simulink library "PUD_lib"  (Simulink 7.5)
settings: Solver=ode45  StartTime=0.0  StopTime=10.0  RelTol=1e-3
values from neighbouring files (symbols this model uses):
  pPUD_cnt_ACChItErrThd_C = Simulink.Parameter    [PUD_par.m]
  pPUD_cnt_ACHeatItErrThd_C = Simulink.Parameter    [PUD_par.m]
  pPUD_cnt_DCChItErrThd_C = Simulink.Parameter    [PUD_par.m]
  pPUD_cnt_DCHeatItErrThd_C = Simulink.Parameter    [PUD_par.m]
  pPUD_s_ACChrg1NoRespTiout_C = Simulink.Parameter    [PUD_par.m]
  pPUD_s_ACChrg2NoRespTiout_C = Simulink.Parameter    [PUD_par.m]
  pPUD_s_ACChrgPtcEnDly_C = Simulink.Parameter    [PUD_par.m]
  pPUD_s_BMSOnNoRespTiout_C = Simulink.Parameter    [PUD_par.m]
  pPUD_s_DCChrg1NoRespTiout_C = Simulink.Parameter    [PUD_par.m]
  pPUD_s_DCChrg2NoRespTiout_C = Simulink.Parameter    [PUD_par.m]
  pPUD_s_EgyCoorrChItRecoverDly_C = Simulink.Parameter    [PUD_par.m]
  pPUD_s_EgyCoorrDlyRstCtr_C = Simulink.Parameter    [PUD_par.m]
  pPUD_s_EgyCoorrNoRespTiout_C = Simulink.Parameter    [PUD_par.m]
  pPUD_V_MotPwrVolt_C = Simulink.Parameter    [PUD_par.m]
  pPUD_V_MotRpdDisVolt_C = Simulink.Parameter    [PUD_par.m]
libraries: BaseOperationLib_Browser x22, PES_CZ_FAW x7, simulink x1
settings Model: Creator=wuaibin  LastModifiedBy=wuaibin

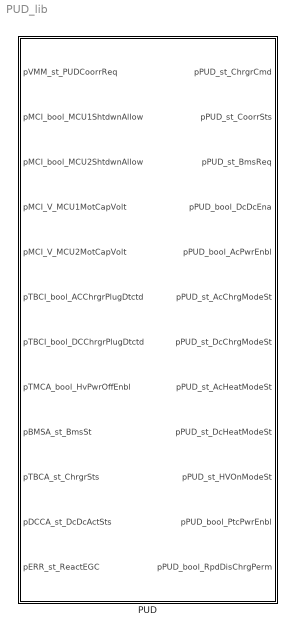
== system PUD_lib ==
  PUD : Subsystem  TreatAsAtomicUnit=on

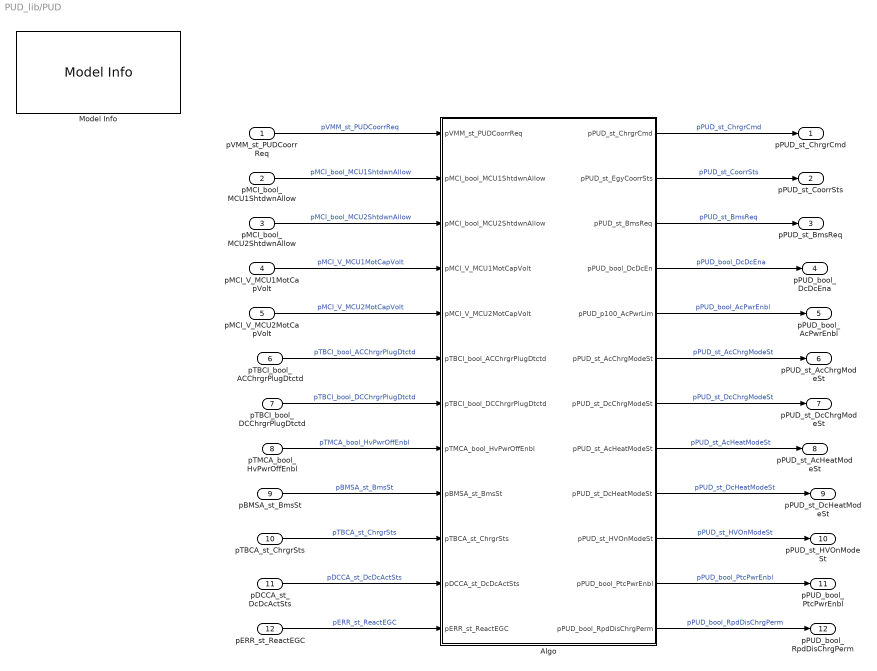
== system PUD_lib/PUD ==
  pVMM_st_PUDCoorrReq : Inport
  pMCI_bool_MCU1ShtdwnAllow : Inport  Port=2
  pMCI_bool_MCU2ShtdwnAllow : Inport  Port=3
  pMCI_V_MCU1MotCapVolt : Inport  Port=4
  pMCI_V_MCU2MotCapVolt : Inport  Port=5
  pTBCI_bool_ACChrgrPlugDtctd : Inport  Port=6
  pTBCI_bool_DCChrgrPlugDtctd : Inport  Port=7
  pTMCA_bool_HvPwrOffEnbl : Inport  Port=8
  pBMSA_st_BmsSt : Inport  Port=9
  pTBCA_st_ChrgrSts : Inport  Port=10
  pDCCA_st_DcDcActSts : Inport  Port=11
  pERR_st_ReactEGC : Inport  Port=12
  Algo : Subsystem
  Model Info : simulink/Model-Wide Utilities/Model Info  SystemSampleTime=-1  InitialBlockCM=None  BlockCM=None  Frame=on  DisplayStringWithTags=Model Info\nCreated: %<Created>\nCreator: wuaibin  HorizontalTextAlignment=Center  LeftAlignmentValue=0.5  SourceBlockDiagram=HQEV_HCU  TagMaxNumber=20
  pPUD_st_ChrgrCmd : Outport
  pPUD_st_CoorrSts : Outport  Port=2
  pPUD_st_BmsReq : Outport  Port=3
  pPUD_bool_DcDcEna : Outport  Port=4
  pPUD_bool_AcPwrEnbl : Outport  Port=5
  pPUD_st_AcChrgModeSt : Outport  Port=6
  pPUD_st_DcChrgModeSt : Outport  Port=7
  pPUD_st_AcHeatModeSt : Outport  Port=8
  pPUD_st_DcHeatModeSt : Outport  Port=9
  pPUD_st_HVOnModeSt : Outport  Port=10
  pPUD_bool_PtcPwrEnbl : Outport  Port=11
  pPUD_bool_RpdDisChrgPerm : Outport  Port=12
  wires:
  pERR_st_ReactEGC/1 -> Algo/12(pERR_st_ReactEGC)  "pERR_st_ReactEGC"
  Algo/12(pPUD_bool_RpdDisChrgPerm) -> pPUD_bool_RpdDisChrgPerm/1  "pPUD_bool_RpdDisChrgPerm"
  pMCI_V_MCU2MotCapVolt/1 -> Algo/5(pMCI_V_MCU2MotCapVolt)  "pMCI_V_MCU2MotCapVolt"
  pMCI_V_MCU1MotCapVolt/1 -> Algo/4(pMCI_V_MCU1MotCapVolt)  "pMCI_V_MCU1MotCapVolt"
  Algo/11(pPUD_bool_PtcPwrEnbl) -> pPUD_bool_PtcPwrEnbl/1  "pPUD_bool_PtcPwrEnbl"
  Algo/10(pPUD_st_HVOnModeSt) -> pPUD_st_HVOnModeSt/1  "pPUD_st_HVOnModeSt"
  Algo/9(pPUD_st_DcHeatModeSt) -> pPUD_st_DcHeatModeSt/1  "pPUD_st_DcHeatModeSt"
  Algo/8(pPUD_st_AcHeatModeSt) -> pPUD_st_AcHeatModeSt/1  "pPUD_st_AcHeatModeSt"
  Algo/7(pPUD_st_DcChrgModeSt) -> pPUD_st_DcChrgModeSt/1  "pPUD_st_DcChrgModeSt"
  Algo/6(pPUD_st_AcChrgModeSt) -> pPUD_st_AcChrgModeSt/1  "pPUD_st_AcChrgModeSt"
  Algo/5(pPUD_p100_AcPwrLim) -> pPUD_bool_AcPwrEnbl/1  "pPUD_bool_AcPwrEnbl"
  Algo/4(pPUD_bool_DcDcEn) -> pPUD_bool_DcDcEna/1  "pPUD_bool_DcDcEna"
  Algo/3(pPUD_st_BmsReq) -> pPUD_st_BmsReq/1  "pPUD_st_BmsReq"
  Algo/2(pPUD_st_EgyCoorrSts) -> pPUD_st_CoorrSts/1  "pPUD_st_CoorrSts"
  Algo/1(pPUD_st_ChrgrCmd) -> pPUD_st_ChrgrCmd/1  "pPUD_st_ChrgrCmd"
  pDCCA_st_DcDcActSts/1 -> Algo/11(pDCCA_st_DcDcActSts)  "pDCCA_st_DcDcActSts"
  pTBCA_st_ChrgrSts/1 -> Algo/10(pTBCA_st_ChrgrSts)  "pTBCA_st_ChrgrSts"
  pBMSA_st_BmsSt/1 -> Algo/9(pBMSA_st_BmsSt)  "pBMSA_st_BmsSt"
  pTMCA_bool_HvPwrOffEnbl/1 -> Algo/8(pTMCA_bool_HvPwrOffEnbl)  "pTMCA_bool_HvPwrOffEnbl"
  pMCI_bool_MCU2ShtdwnAllow/1 -> Algo/3(pMCI_bool_MCU2ShtdwnAllow)  "pMCI_bool_MCU2ShtdwnAllow"
  pMCI_bool_MCU1ShtdwnAllow/1 -> Algo/2(pMCI_bool_MCU1ShtdwnAllow)  "pMCI_bool_MCU1ShtdwnAllow"
  pVMM_st_PUDCoorrReq/1 -> Algo/1(pVMM_st_PUDCoorrReq)  "pVMM_st_PUDCoorrReq"
  pTBCI_bool_ACChrgrPlugDtctd/1 -> Algo/6(pTBCI_bool_ACChrgrPlugDtctd)  "pTBCI_bool_ACChrgrPlugDtctd"
  pTBCI_bool_DCChrgrPlugDtctd/1 -> Algo/7(pTBCI_bool_DCChrgrPlugDtctd)  "pTBCI_bool_DCChrgrPlugDtctd"

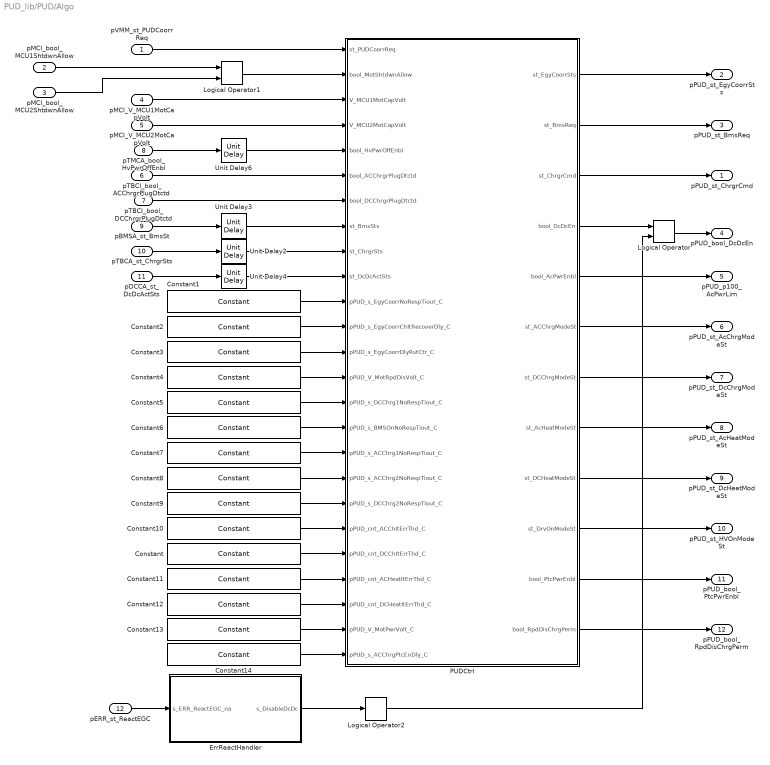
== system PUD_lib/PUD/Algo ==
  pVMM_st_PUDCoorrReq : Inport
  pMCI_bool_MCU1ShtdwnAllow : Inport  Port=2
  pMCI_bool_MCU2ShtdwnAllow : Inport  Port=3
  pMCI_V_MCU1MotCapVolt : Inport  Port=4
  pMCI_V_MCU2MotCapVolt : Inport  Port=5
  pTBCI_bool_ACChrgrPlugDtctd : Inport  Port=6
  pTBCI_bool_DCChrgrPlugDtctd : Inport  Port=7
  pTMCA_bool_HvPwrOffEnbl : Inport  Port=8
  pBMSA_st_BmsSt : Inport  Port=9
  pTBCA_st_ChrgrSts : Inport  Port=10
  pDCCA_st_DcDcActSts : Inport  Port=11
  pERR_st_ReactEGC : Inport  Port=12
  Constant : BaseOperationLib_Browser/Sources&Sinks/Constant  Value=pPUD_cnt_DCChItErrThd_C  OutMin=[]  OutMax=[]  OutDataType=fixdt(1, 16)  ConRadixGroup=Use specified scaling  OutScaling=2^0  OutDataTypeStr=Inherit: Inherit from 'Constant value'
  Constant1 : BaseOperationLib_Browser/Sources&Sinks/Constant  Value=pPUD_s_EgyCoorrNoRespTiout_C  OutMin=[]  OutMax=[]  OutDataType=fixdt(1, 16)  ConRadixGroup=Use specified scaling  OutScaling=2^0  OutDataTypeStr=Inherit: Inherit from 'Constant value'
  Constant10 : BaseOperationLib_Browser/Sources&Sinks/Constant  Value=pPUD_cnt_ACChItErrThd_C  OutMin=[]  OutMax=[]  OutDataType=fixdt(1, 16)  ConRadixGroup=Use specified scaling  OutScaling=2^0  OutDataTypeStr=Inherit: Inherit from 'Constant value'
  Constant11 : BaseOperationLib_Browser/Sources&Sinks/Constant  Value=pPUD_cnt_ACHeatItErrThd_C  OutMin=[]  OutMax=[]  OutDataType=fixdt(1, 16)  ConRadixGroup=Use specified scaling  OutScaling=2^0  OutDataTypeStr=Inherit: Inherit from 'Constant value'
  Constant12 : BaseOperationLib_Browser/Sources&Sinks/Constant  Value=pPUD_cnt_DCHeatItErrThd_C  OutMin=[]  OutMax=[]  OutDataType=fixdt(1, 16)  ConRadixGroup=Use specified scaling  OutScaling=2^0  OutDataTypeStr=Inherit: Inherit from 'Constant value'
  Constant13 : BaseOperationLib_Browser/Sources&Sinks/Constant  Value=pPUD_V_MotPwrVolt_C  OutMin=[]  OutMax=[]  OutDataType=fixdt(1, 16)  ConRadixGroup=Use specified scaling  OutScaling=2^0  OutDataTypeStr=Inherit: Inherit from 'Constant value'
  Constant14 : BaseOperationLib_Browser/Sources&Sinks/Constant  Value=pPUD_s_ACChrgPtcEnDly_C  OutMin=[]  OutMax=[]  OutDataType=fixdt(1, 16)  ConRadixGroup=Use specified scaling  OutScaling=2^0  OutDataTypeStr=Inherit: Inherit from 'Constant value'
  Constant2 : BaseOperationLib_Browser/Sources&Sinks/Constant  Value=pPUD_s_EgyCoorrChItRecoverDly_C  OutMin=[]  OutMax=[]  OutDataType=fixdt(1, 16)  ConRadixGroup=Use specified scaling  OutScaling=2^0  OutDataTypeStr=Inherit: Inherit from 'Constant value'
  Constant3 : BaseOperationLib_Browser/Sources&Sinks/Constant  Value=pPUD_s_EgyCoorrDlyRstCtr_C  OutMin=[]  OutMax=[]  OutDataType=fixdt(1, 16)  ConRadixGroup=Use specified scaling  OutScaling=2^0  OutDataTypeStr=Inherit: Inherit from 'Constant value'
  Constant4 : BaseOperationLib_Browser/Sources&Sinks/Constant  Value=pPUD_V_MotRpdDisVolt_C  OutMin=[]  OutMax=[]  OutDataType=fixdt(1, 16)  ConRadixGroup=Use specified scaling  OutScaling=2^0  OutDataTypeStr=Inherit: Inherit from 'Constant value'
  Constant5 : BaseOperationLib_Browser/Sources&Sinks/Constant  Value=pPUD_s_DCChrg1NoRespTiout_C  OutMin=[]  OutMax=[]  OutDataType=fixdt(1, 16)  ConRadixGroup=Use specified scaling  OutScaling=2^0  OutDataTypeStr=Inherit: Inherit from 'Constant value'
  Constant6 : BaseOperationLib_Browser/Sources&Sinks/Constant  Value=pPUD_s_BMSOnNoRespTiout_C  VectorParams1D=off  OutMin=[]  OutMax=[]  OutDataType=fixdt(1, 16)  ConRadixGroup=Use specified scaling  OutScaling=2^0  OutDataTypeStr=Inherit: Inherit from 'Constant value'
  Constant7 : BaseOperationLib_Browser/Sources&Sinks/Constant  Value=pPUD_s_ACChrg1NoRespTiout_C  OutMin=[]  OutMax=[]  OutDataType=fixdt(1, 16)  ConRadixGroup=Use specified scaling  OutScaling=2^0  OutDataTypeStr=Inherit: Inherit from 'Constant value'
  Constant8 : BaseOperationLib_Browser/Sources&Sinks/Constant  Value=pPUD_s_ACChrg2NoRespTiout_C  OutMin=[]  OutMax=[]  OutDataType=fixdt(1, 16)  ConRadixGroup=Use specified scaling  OutScaling=2^0  OutDataTypeStr=Inherit: Inherit from 'Constant value'
  Constant9 : BaseOperationLib_Browser/Sources&Sinks/Constant  Value=pPUD_s_DCChrg2NoRespTiout_C  OutMin=[]  OutMax=[]  OutDataType=fixdt(1, 16)  ConRadixGroup=Use specified scaling  OutScaling=2^0  OutDataTypeStr=Inherit: Inherit from 'Constant value'
  ErrReactHandler : Subsystem
  Logical Operator : BaseOperationLib_Browser/Logic Operations Changed/Logical Operator  Operator=AND  Inputs=2  AllPortsSameDT=off  OutDataTypeMode=boolean  LogicDataType=PDT_Bool  OutDataTypeStr=boolean
  Logical Operator1 : BaseOperationLib_Browser/Logic Operations Changed/Logical Operator  Operator=AND  Inputs=2  AllPortsSameDT=off  OutDataTypeMode=boolean  LogicDataType=PDT_Bool  OutDataTypeStr=boolean
  Logical Operator2 : BaseOperationLib_Browser/Logic Operations Changed/Logical Operator  Operator=NOT  Inputs=2  AllPortsSameDT=off  OutDataTypeMode=boolean  LogicDataType=PDT_Bool  OutDataTypeStr=boolean
  PUDCtrl : Stateflow chart  TreatAsAtomicUnit=on
  Unit Delay{2..4,6} (4 alike) : BaseOperationLib_Browser/Discrete Unchanged /Unit Delay  X0=0  SampleTime=-1
  pPUD_st_ChrgrCmd : Outport
  pPUD_st_EgyCoorrSts : Outport  Port=2
  pPUD_st_BmsReq : Outport  Port=3
  pPUD_bool_DcDcEn : Outport  Port=4
  pPUD_p100_AcPwrLim : Outport  Port=5
  pPUD_st_AcChrgModeSt : Outport  Port=6
  pPUD_st_DcChrgModeSt : Outport  Port=7
  pPUD_st_AcHeatModeSt : Outport  Port=8
  pPUD_st_DcHeatModeSt : Outport  Port=9
  pPUD_st_HVOnModeSt : Outport  Port=10
  pPUD_bool_PtcPwrEnbl : Outport  Port=11
  pPUD_bool_RpdDisChrgPerm : Outport  Port=12
  wires:
  Logical Operator2/1 -> Logical Operator/2
  Constant12/1 -> PUDCtrl/23(pPUD_cnt_DCHeatItErrThd_C)
  Constant11/1 -> PUDCtrl/22(pPUD_cnt_ACHeatItErrThd_C)
  Constant10/1 -> PUDCtrl/20(pPUD_cnt_ACChItErrThd_C)
  Constant9/1 -> PUDCtrl/19(pPUD_s_DCChrg2NoRespTiout_C)
  Constant8/1 -> PUDCtrl/18(pPUD_s_ACChrg2NoRespTiout_C)
  Constant7/1 -> PUDCtrl/17(pPUD_s_ACChrg1NoRespTiout_C)
  Constant6/1 -> PUDCtrl/16(pPUD_s_BMSOnNoRespTiout_C)
  Constant5/1 -> PUDCtrl/15(pPUD_s_DCChrg1NoRespTiout_C)
  Constant4/1 -> PUDCtrl/14(pPUD_V_MotRpdDisVolt_C)
  Constant3/1 -> PUDCtrl/13(pPUD_s_EgyCoorrDlyRstCtr_C)
  Constant2/1 -> PUDCtrl/12(pPUD_s_EgyCoorrChItRecoverDly_C)
  Constant1/1 -> PUDCtrl/11(pPUD_s_EgyCoorrNoRespTiout_C)
  Constant/1 -> PUDCtrl/21(pPUD_cnt_DCChItErrThd_C)
  pERR_st_ReactEGC/1 -> ErrReactHandler/1(s_ERR_ReactEGC_na)
  ErrReactHandler/1(s_DisableDcDc) -> Logical Operator2/1
  Logical Operator/1 -> pPUD_bool_DcDcEn/1
  PUDCtrl/12(bool_RpdDisChrgPerm) -> pPUD_bool_RpdDisChrgPerm/1
  pMCI_V_MCU2MotCapVolt/1 -> PUDCtrl/4(V_MCU2MotCapVolt)
  pMCI_V_MCU1MotCapVolt/1 -> PUDCtrl/3(V_MCU1MotCapVolt)
  Logical Operator1/1 -> PUDCtrl/2(bool_MotShtdwnAllow)
  pMCI_bool_MCU1ShtdwnAllow/1 -> Logical Operator1/1
  pMCI_bool_MCU2ShtdwnAllow/1 -> Logical Operator1/2
  Unit Delay4/1 -> PUDCtrl/10(st_DcDcActSts)
  Unit Delay2/1 -> PUDCtrl/9(st_ChrgrSts)
  Unit Delay3/1 -> PUDCtrl/8(st_BmsSts)
  Unit Delay6/1 -> PUDCtrl/5(bool_HvPwrOffEnbl)
  PUDCtrl/11(bool_PtcPwrEnbl) -> pPUD_bool_PtcPwrEnbl/1
  PUDCtrl/10(st_DrvOnModeSt) -> pPUD_st_HVOnModeSt/1
  PUDCtrl/9(st_DCHeatModeSt) -> pPUD_st_DcHeatModeSt/1
  PUDCtrl/8(st_AcHeatModeSt) -> pPUD_st_AcHeatModeSt/1
  PUDCtrl/7(st_DCChrgModeSt) -> pPUD_st_DcChrgModeSt/1
  PUDCtrl/6(st_ACChrgModeSt) -> pPUD_st_AcChrgModeSt/1
  pTMCA_bool_HvPwrOffEnbl/1 -> Unit Delay6/1
  PUDCtrl/5(bool_AcPwrEnbl) -> pPUD_p100_AcPwrLim/1
  pTBCA_st_ChrgrSts/1 -> Unit Delay2/1
  pBMSA_st_BmsSt/1 -> Unit Delay3/1
  PUDCtrl/3(st_ChrgrCmd) -> pPUD_st_ChrgrCmd/1
  PUDCtrl/2(st_BmsReq) -> pPUD_st_BmsReq/1
  PUDCtrl/1(st_EgyCoorrSts) -> pPUD_st_EgyCoorrSts/1
  pVMM_st_PUDCoorrReq/1 -> PUDCtrl/1(st_PUDCoorrReq)
  pDCCA_st_DcDcActSts/1 -> Unit Delay4/1
  PUDCtrl/4(bool_DcDcEn) -> Logical Operator/1
  pTBCI_bool_ACChrgrPlugDtctd/1 -> PUDCtrl/6(bool_ACChrgrPlugDtctd)
  pTBCI_bool_DCChrgrPlugDtctd/1 -> PUDCtrl/7(bool_DCChrgrPlugDtctd)
  Constant13/1 -> PUDCtrl/24(pPUD_V_MotPwrVolt_C)
  Constant14/1 -> PUDCtrl/25(pPUD_s_ACChrgPtcEnDly_C)

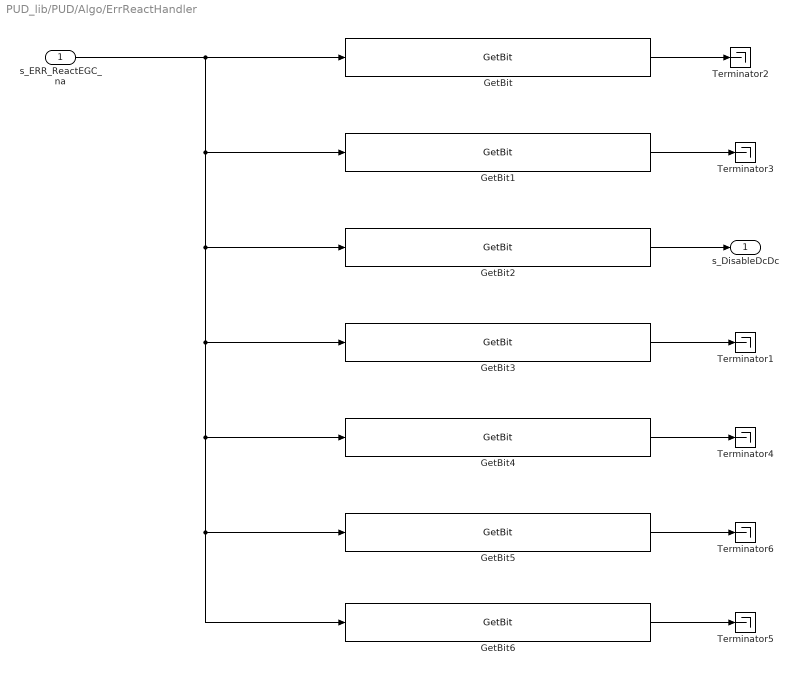
== system PUD_lib/PUD/Algo/ErrReactHandler ==
  s_ERR_ReactEGC_na : Inport
  GetBit : PES_CZ_FAW/Discontinuities/GetBit  SystemSampleTime=-1  maska=FtlReactEGCTyp.POWER_LIMIT
  GetBit1 : PES_CZ_FAW/Discontinuities/GetBit  SystemSampleTime=-1  maska=FtlReactEGCTyp.EMERGENCY_HV_OFF
  GetBit2 : PES_CZ_FAW/Discontinuities/GetBit  SystemSampleTime=-1  maska=FtlReactEGCTyp.NO_LV_CHARGING
  GetBit3 : PES_CZ_FAW/Discontinuities/GetBit  SystemSampleTime=-1  maska=FtlReactEGCTyp.LV_ACCESSORY_REDUCTION
  GetBit4 : PES_CZ_FAW/Discontinuities/GetBit  SystemSampleTime=-1  maska=FtlReactEGCTyp.NO_HVDC_CHARGING
  GetBit5 : PES_CZ_FAW/Discontinuities/GetBit  SystemSampleTime=-1  maska=FtlReactEGCTyp.REPEAT_CHARGING_ATTEMPT
  GetBit6 : PES_CZ_FAW/Discontinuities/GetBit  SystemSampleTime=-1  maska=FtlReactEGCTyp.NO_HV_CHARGING
  Terminator{1..6} (6 alike) : Terminator
  s_DisableDcDc : Outport
  wires:
  GetBit5/1 -> Terminator6/1
  GetBit1/1 -> Terminator3/1
  s_ERR_ReactEGC_na/1 -> GetBit1/1, GetBit2/1, GetBit3/1, GetBit4/1, GetBit6/1, GetBit5/1, GetBit/1
  GetBit6/1 -> Terminator5/1
  GetBit4/1 -> Terminator4/1
  GetBit3/1 -> Terminator1/1
  GetBit/1 -> Terminator2/1
  GetBit2/1 -> s_DisableDcDc/1

== stateflow chart PUD/Algo/PUDCtrl ==
  state EmgHVOff
    en:
    st_EgyCoorrSts = PUDCoorrStsTyp.PUD_EmgHVOFF;
    settings: description=Irrecoverable error state. This state is entered from any other state in the case of irrecoverable error and can only be left back into the HVoff state by resetting Clamp15 (ignition).
    state HVOFF_OK
      en:
      st_EgyCoorrSts = PUDCoorrStsTyp.PUD_EmgHVOFF_OK;
    state BMS_HVOFF
      en:
      st_BmsReq = BMSCmdTyp.BMS_CMD_EmgHVOFF;
    state RapidDischarge
      entry:
      bool_RpdDisChrgPerm = true;
    state HvOff_ERR
      entry:
      st_EgyCoorrSts = PUDCoorrStsTyp.PUD_EmgHVOFF_ERR;
    state Motor_STOP
      entry:
      bool_DcDcEn = false;
      bool_AcPwrEnbl = false;
      bool_PtcPwrEnbl = false;
      st_ChrgrCmd = ChrgrCmdTyp.STOP;
    EmgHVOff.HvOff_ERR -> HVOFF_OK : [V_MCU1MotCapVolt < pPUD_V_MotRpdDisVolt_C && ...
        | V_MCU2MotCapVolt < pPUD_V_MotRpdDisVolt_C ]
    EmgHVOff.RapidDischarge -> HVOFF_OK : [V_MCU1MotCapVolt < pPUD_V_MotRpdDisVolt_C && ...
        | V_MCU2MotCapVolt < pPUD_V_MotRpdDisVolt_C ]
    (default) -> Motor_STOP
    BMS_HVOFF -> EmgHVOff.HvOff_ERR [order 2] : [st_BmsSts == BMSStsTyp.BMS_EmgHVOFF_ERR]
    BMS_HVOFF -> EmgHVOff.RapidDischarge [order 1] : [st_BmsSts == BMSStsTyp.BMS_EmgHVOFF_OK]
    Motor_STOP -> BMS_HVOFF
  state Normal
    state ACChrg
      state ACChrg
        settings: description=Charging control superstate.
        state BmsOkDcDcOnAcOn
          entry:
          bool_DcDcEn = true;
          bool_AcPwrEnbl = true;
        state ACChrgPhase2
          entry:
          st_ChrgrCmd = uint8(ChrgrCmdTyp.ACChrg_PHASE2);
        state ChrgCheck
          entry:
          st_ChrgrCmd = uint8(ChrgrCmdTyp.ACChrg_PHASE1);
        state BmsACChrgOn
          entry:
          st_BmsReq = uint8(BMSCmdTyp.BMS_CMD_ACChrgOn);
        state ACChargingInterrupted
          entry:
          ChItCtr = ChItCtr + 1;
          bool_DcDcEn = false;
          bool_AcPwrEnbl = false;
          bool_PtcPwrEnbl = false;
          st_ChrgrCmd = uint8(ChrgrCmdTyp.STOP);
        state ChrgInit
        state ACCharging
          settings: description=Charging control superstate.
          state Charging
            entry:
            st_ACChrgModeSt = ACChrgModeTyp.PUD_ACChrg_On;
            st_EgyCoorrSts = PUDCoorrStsTyp.PUD_ACChrgOn;
            settings: description=Normal charging operation. Charger mains maximum current and target voltage are set and charger is commanded to Active state on entry. Charger output current is computed dynamically according current BMS charging limitations. Start of charging is indicated acoustically by the buzzer.
          (default) -> Normal.ACChrg.ACChrg.ACCharging.Charging
          ACCharging -> ACCharging [order 1] : after(pPUD_s_EgyCoorrDlyRstCtr_C,sec)/ChItCtr = 0;
        ACCharging -> ACChargingInterrupted [order 1] : [st_ChrgrSts == ChrgrStsTyp.CST_STOP]
        BmsACChrgOn -> Normal.ACChrg.ACChrg.BmsOkDcDcOnAcOn [order 1] : [st_BmsSts == BMSStsTyp.BMS_ACChrgOn]
        Normal.ACChrg.ACChrg.BmsOkDcDcOnAcOn -> ACChargingInterrupted [order 2] : after(pPUD_s_EgyCoorrNoRespTiout_C,sec)
        ACChrgPhase2 -> ACCharging [order 1] : [st_ChrgrSts == ChrgrStsTyp.CST_ACChrg_PHASE2]
        ACChrgPhase2 -> ACChargingInterrupted [order 2] : after(pPUD_s_ACChrg2NoRespTiout_C,sec)
        Normal.ACChrg.ACChrg.BmsOkDcDcOnAcOn -> ACChrgPhase2 [order 1] : [st_DcDcActSts == DCDCAStsTyp.DST_Working]
        BmsACChrgOn -> ACChargingInterrupted [order 2] : after(pPUD_s_EgyCoorrNoRespTiout_C,sec)
        (default) -> ChrgInit
        ACChargingInterrupted -> ChrgInit : after(pPUD_s_EgyCoorrChItRecoverDly_C,sec)
        ChrgInit -> ChrgCheck
        ChrgCheck -> ACChargingInterrupted [order 2] : after(pPUD_s_ACChrg1NoRespTiout_C,sec)
        ChrgCheck -> BmsACChrgOn [order 1] : [st_ChrgrSts == ChrgrStsTyp.CST_ACChrg_PHASE1]
      state Init
        entry:
        st_ChrgrCmd = ChrgrCmdTyp.STOP;
        bool_DcDcEn = false;
        bool_AcPwrEnbl = false;
        bool_PtcPwrEnbl = false;
        ChItCtr = 0;
        SlaveNoResponse = 0;
        st_ACChrgModeSt = ACChrgModeTyp.PUD_ACChrg_Init;
      state ACChrgError
        entry:
        st_ACChrgModeSt = ACChrgModeTyp.PUD_ACChrg_Err;
        settings: description=Irrecoverable error state. This state is entered from any other state in the case of irrecoverable error and can only be left back into the HVoff state by resetting Clamp15 (ignition).
      Normal.ACChrg.Init -> Normal.ACChrg.ACChrg
      Normal.ACChrg.ACChrg -> ACChrgError : [ChItCtr > pPUD_cnt_ACChItErrThd_C]
      (default) -> Normal.ACChrg.Init
    state Init
      entry:
      ChItCtr = 0;
      SlaveNoResponse = 0;
      st_ACChrgModeSt = 0;
      st_DCChrgModeSt = 0;
      st_AcHeatModeSt = 0;
      st_DCHeatModeSt = 0;
      st_DrvOnModeSt = 0;
      bool_DcDcEn = false;
      bool_AcPwrEnbl = false;
      bool_PtcPwrEnbl = false;
      st_ChrgrCmd = ChrgrCmdTyp.IDLE;
      st_EgyCoorrSts = PUDCoorrStsTyp.PUD_Init;
      settings: description=HV off state. BMS is in HVoff or Shutdown state, depending on the operation mode (clamp status). If ignition is off the BMS is commanded to shutdown, if ignition is on it only goes to HVoff. This decision is made in the SetBMSCmd function.
    state Drv
      exit:
      st_DrvOnModeSt = DrvOnModeTyp.PUD_DrvOn_Init;
      settings: description=BMS HVon state.
      state DrvOn
        state DrvOn_Err
          entry:
          st_DrvOnModeSt = DrvOnModeTyp.PUD_DrvOn_Err;
          settings: description=Irrecoverable error state. This state is entered from any other state in the case of irrecoverable error and can only be left back into the HVoff state by resetting Clamp15 (ignition).
        state DrvOn_Init
          entry:
          st_ChrgrCmd = ChrgrCmdTyp.STOP;
          bool_DcDcEn = false;
          bool_AcPwrEnbl = false;
          bool_PtcPwrEnbl = false;
          ChItCtr = 0;
          SlaveNoResponse = 0;
          st_DrvOnModeSt = DrvOnModeTyp.PUD_DrvOn_Init;
        state DrvOn_On
          en:
          st_EgyCoorrSts = PUDCoorrStsTyp.PUD_DrvOn;
          state HvOn
            entry:
            st_DrvOnModeSt = DrvOnModeTyp.PUD_DrvOn_Ok;
            st_EgyCoorrSts = PUDCoorrStsTyp.PUD_DrvOn;
          state BMSOn
            entry:
            st_BmsReq = uint8(BMSCmdTyp.BMS_CMD_HVOn);
          state BmsOk_DcDcOnAcOn
            entry:
            bool_DcDcEn = true;
            bool_AcPwrEnbl = true;
            bool_PtcPwrEnbl = true;
          state ChargerInit
          state HvOn_Failed
            entry:
            ChItCtr = ChItCtr + 1;
            st_ChrgrCmd = uint8(ChrgrCmdTyp.STOP);
          (default) -> Normal.Drv.DrvOn.DrvOn_On.ChargerInit
          Normal.Drv.DrvOn.DrvOn_On.ChargerInit -> BMSOn
          BMSOn -> HvOn_Failed [order 2] : after(pPUD_s_EgyCoorrNoRespTiout_C,sec)
          BMSOn -> BmsOk_DcDcOnAcOn [order 1] : [st_BmsSts == BMSStsTyp.BMS_HVOn]
          BmsOk_DcDcOnAcOn -> HvOn
        DrvOn_Init -> DrvOn_On
        DrvOn_On -> DrvOn_Err : [ChItCtr > 0]
        (default) -> DrvOn_Init
      state DrvErr
        state Motor_ShtDwn
        state Init
          entry:
          bool_DcDcEn = false;
          bool_AcPwrEnbl = false;
          bool_PtcPwrEnbl = false;
          ChItCtr = 0;
          SlaveNoResponse = 0;
        state HvOff
          entry:
          st_EgyCoorrSts = PUDCoorrStsTyp.PUD_DrvErr;
        state DcDcOffOk_BmsOffAcOff
          entry:
          st_BmsReq = uint8(BMSCmdTyp.BMS_CMD_HVOFF);
        DcDcOffOk_BmsOffAcOff -> Normal.Drv.DrvErr.HvOff : [st_BmsSts == BMSStsTyp.BMS_HVOFF_OK]
        Normal.Drv.DrvErr.Init -> Normal.Drv.DrvErr.Motor_ShtDwn : [st_DcDcActSts ==DCDCAStsTyp.DST_ShutDown && ...
            | bool_HvPwrOffEnbl == true || ...
            | after(pPUD_s_EgyCoorrNoRespTiout_C,sec)]
        (default) -> Normal.Drv.DrvErr.Init
        Normal.Drv.DrvErr.Motor_ShtDwn -> DcDcOffOk_BmsOffAcOff : [bool_MotShtdwnAllow == true]
      DrvErr -> DrvOn : [st_PUDCoorrReq == PUDCoorrStsTyp.PUD_DrvOn]
      DrvOn -> DrvErr : [st_PUDCoorrReq == PUDCoorrStsTyp.PUD_DrvErr]
      (default) -> DrvOn
    state DCChrg
      settings: description=Charging control superstate.
      state DCChrg_On
        settings: description=Charging control superstate.
        state DCChrging
          settings: description=Charging control superstate.
          state Charging
            entry:
            st_DCChrgModeSt = DCChrgModeTyp.PUD_DCChrg_On;
            st_EgyCoorrSts = PUDCoorrStsTyp.PUD_DCChrgOn;
            settings: description=Normal charging operation. Charger mains maximum current and target voltage are set and charger is commanded to Active state on entry. Charger output current is computed dynamically according current BMS charging limitations. Start of charging is indicated acoustically by the buzzer.
          DCChrging -> DCChrging [order 1] : after(pPUD_s_EgyCoorrDlyRstCtr_C,sec)/ChItCtr = 0;
          (default) -> Normal.DCChrg.DCChrg_On.DCChrging.Charging
        state BmsOkDcDcOnAcOn
          entry:
          bool_DcDcEn = true;
          bool_AcPwrEnbl = true;
        state DCChrgPhase2
          entry:
          st_ChrgrCmd = uint8(ChrgrCmdTyp.DCChrg_PHASE2);
        state BmsDCChrgOn
          entry:
          st_BmsReq = uint8(BMSCmdTyp.BMS_CMD_DCChrgOn);
        state ChargerInit
        state ChargingInterrupted
          entry:
          ChItCtr = ChItCtr + 1;
          bool_DcDcEn = false;
          bool_AcPwrEnbl = false;
          bool_PtcPwrEnbl = false;
          st_ChrgrCmd = uint8(ChrgrCmdTyp.STOP);
        state DCChrgPhase1
          entry:
          st_ChrgrCmd = uint8(ChrgrCmdTyp.DCChrg_PHASE1);
        DCChrging -> Normal.DCChrg.DCChrg_On.ChargingInterrupted [order 1] : [st_ChrgrSts == ChrgrStsTyp.CST_STOP]
        DCChrgPhase2 -> DCChrging [order 1] : [st_ChrgrSts == ChrgrStsTyp.CST_DCChrg_PHASE2]
        DCChrgPhase2 -> Normal.DCChrg.DCChrg_On.ChargingInterrupted [order 2] : after(pPUD_s_DCChrg2NoRespTiout_C,sec)
        Normal.DCChrg.DCChrg_On.BmsOkDcDcOnAcOn -> DCChrgPhase2 [order 1] : [st_DcDcActSts == DCDCAStsTyp.DST_Working]
        Normal.DCChrg.DCChrg_On.BmsOkDcDcOnAcOn -> Normal.DCChrg.DCChrg_On.ChargingInterrupted [order 2] : after(pPUD_s_EgyCoorrNoRespTiout_C,sec)
        BmsDCChrgOn -> Normal.DCChrg.DCChrg_On.BmsOkDcDcOnAcOn [order 1] : [st_BmsSts == BMSStsTyp.BMS_DCChrgOn]
        BmsDCChrgOn -> Normal.DCChrg.DCChrg_On.ChargingInterrupted [order 2] : after(pPUD_s_EgyCoorrNoRespTiout_C,sec)
        DCChrgPhase1 -> BmsDCChrgOn [order 2] : [st_ChrgrSts == ChrgrStsTyp.CST_DCChrg_PHASE1]
        DCChrgPhase1 -> Normal.DCChrg.DCChrg_On.ChargingInterrupted [order 1] : after(pPUD_s_DCChrg1NoRespTiout_C,sec)
        Normal.DCChrg.DCChrg_On.ChargerInit -> DCChrgPhase1
        Normal.DCChrg.DCChrg_On.ChargingInterrupted -> Normal.DCChrg.DCChrg_On.ChargerInit : after(pPUD_s_EgyCoorrChItRecoverDly_C,sec)
        (default) -> Normal.DCChrg.DCChrg_On.ChargerInit
      state DCChrg_Err
        entry:
        st_DCChrgModeSt = DCChrgModeTyp.PUD_DCChrg_Err;
        settings: description=Irrecoverable error state. This state is entered from any other state in the case of irrecoverable error and can only be left back into the HVoff state by resetting Clamp15 (ignition).
      state DCChrg_Init
        entry:
        st_ChrgrCmd = ChrgrCmdTyp.STOP;
        st_DCChrgModeSt = DCChrgModeTyp.PUD_DCChrg_Init;
        bool_DcDcEn = false;
        bool_AcPwrEnbl = false;
        bool_PtcPwrEnbl = false;
        ChItCtr = 0;
        SlaveNoResponse = 0;
      DCChrg_Init -> DCChrg_On
      (default) -> DCChrg_Init
      DCChrg_On -> DCChrg_Err : [ChItCtr > pPUD_cnt_DCChItErrThd_C]
    state ACHeat
      state ACHeat_Init
        entry:
        st_ChrgrCmd = ChrgrCmdTyp.STOP;
        bool_DcDcEn = false;
        bool_AcPwrEnbl = false;
        bool_PtcPwrEnbl = false;
        st_AcHeatModeSt = ACHeatModeTyp.PUD_ACHeat_Init;
        ChItCtr = 0;
        SlaveNoResponse = 0;
      state ACHeat_On
        settings: description=Charging control superstate.
        state PtcEna
          entry:
          bool_PtcPwrEnbl = true;
        state ACHeating
          settings: description=Charging control superstate.
          state Heating
            entry:
            st_AcHeatModeSt = ACHeatModeTyp.PUD_ACHeat_On;
            st_EgyCoorrSts = PUDCoorrStsTyp.PUD_ACHeatOn;
            settings: description=Normal charging operation. Charger mains maximum current and target voltage are set and charger is commanded to Active state on entry. Charger output current is computed dynamically according current BMS charging limitations. Start of charging is indicated acoustically by the buzzer.
          (default) -> Normal.ACHeat.ACHeat_On.ACHeating.Heating
          ACHeating -> ACHeating [order 1] : after(pPUD_s_EgyCoorrDlyRstCtr_C,sec)/ChItCtr = 0;
        state ACHeatPhase2
          entry:
          st_ChrgrCmd = uint8(ChrgrCmdTyp.ACHeat_PHASE2);
        state DcDcEna
          entry:
          bool_DcDcEn = true;
        state ChargingInterrupted
          entry:
          ChItCtr = ChItCtr + 1;
          bool_DcDcEn = false;
          bool_PtcPwrEnbl = false;
          bool_AcPwrEnbl = false;
          st_ChrgrCmd = ChrgrCmdTyp.STOP;
        state ACHeatPhase1
          entry:
          st_ChrgrCmd = ChrgrCmdTyp.ACHeat_PHASE1;
        state HVOFF
          entry:
          st_BmsReq = uint8(BMSCmdTyp.BMS_CMD_HVOFF);
        state ChargerInit
        state BmsACHeatOn
          entry:
          st_BmsReq = uint8(BMSCmdTyp.BMS_CMD_ACHeatOn);
        Normal.ACHeat.ACHeat_On.HVOFF -> ACHeatPhase2 [order 2] : [st_BmsSts == BMSStsTyp.BMS_HVOFF_OK]
        BmsACHeatOn -> Normal.ACHeat.ACHeat_On.ChargingInterrupted [order 2] : after(pPUD_s_EgyCoorrNoRespTiout_C,sec)
        ACHeatPhase1 -> Normal.ACHeat.ACHeat_On.ChargingInterrupted [order 1] : after(pPUD_s_ACChrg1NoRespTiout_C,sec)
        DcDcEna -> ACHeating [order 2] : [st_DcDcActSts == DCDCAStsTyp.DST_Working]
        DcDcEna -> Normal.ACHeat.ACHeat_On.ChargingInterrupted [order 1] : after(pPUD_s_EgyCoorrNoRespTiout_C,sec)
        ACHeatPhase2 -> BmsACHeatOn [order 2] : [st_ChrgrSts == ChrgrStsTyp.CST_ACHeat_PHASE2]
        ACHeatPhase2 -> Normal.ACHeat.ACHeat_On.ChargingInterrupted [order 1] : after(pPUD_s_ACChrg2NoRespTiout_C,sec)
        BmsACHeatOn -> PtcEna [order 1] : [st_BmsSts == BMSStsTyp.BMS_ACHeatOn]
        Normal.ACHeat.ACHeat_On.HVOFF -> Normal.ACHeat.ACHeat_On.ChargingInterrupted [order 1] : after(pPUD_s_EgyCoorrNoRespTiout_C,sec)
        (default) -> Normal.ACHeat.ACHeat_On.ChargerInit
        ACHeating -> Normal.ACHeat.ACHeat_On.ChargingInterrupted [order 1] : [st_ChrgrSts == ChrgrStsTyp.CST_STOP]
        Normal.ACHeat.ACHeat_On.ChargerInit -> ACHeatPhase1
        ACHeatPhase1 -> Normal.ACHeat.ACHeat_On.HVOFF [order 2] : [st_ChrgrSts == ChrgrStsTyp.CST_ACHeat_PHASE1]
        Normal.ACHeat.ACHeat_On.ChargingInterrupted -> Normal.ACHeat.ACHeat_On.ChargerInit : after(pPUD_s_EgyCoorrChItRecoverDly_C,sec)
        PtcEna -> DcDcEna [order 1] : [after(pPUD_s_ACChrgPtcEnDly_C,sec) && ...
            |  V_MCU1MotCapVolt > pPUD_V_MotPwrVolt_C]
        PtcEna -> Normal.ACHeat.ACHeat_On.ChargingInterrupted [order 2] : [after(pPUD_s_ACChrgPtcEnDly_C,sec) && ...
            |  V_MCU1MotCapVolt < pPUD_V_MotPwrVolt_C]
      state ACHeat_Error
        entry:
        st_AcHeatModeSt = ACHeatModeTyp.PUD_ACHeat_Err;
        settings: description=Irrecoverable error state. This state is entered from any other state in the case of irrecoverable error and can only be left back into the HVoff state by resetting Clamp15 (ignition).
      ACHeat_On -> ACHeat_Error : [ChItCtr > pPUD_cnt_ACHeatItErrThd_C]
      ACHeat_Init -> ACHeat_On
      (default) -> ACHeat_Init
    state HVOff
      entry:
      st_EgyCoorrSts = PUDCoorrStsTyp.PUD_HVOFF;
      settings: description=HV off state. BMS is in HVoff or Shutdown state, depending on the operation mode (clamp status). If ignition is off the BMS is commanded to shutdown, if ignition is on it only goes to HVoff. This decision is made in the SetBMSCmd function.
      state HV_OFF [parallel]
        settings: executionOrder=1
        state HvOff
          entry:
          st_EgyCoorrSts = PUDCoorrStsTyp.PUD_HVOFF_OK;
        state HvOff_ERR
          entry:
          st_EgyCoorrSts = PUDCoorrStsTyp.PUD_HVOFF_ERR;
        state RapidDischarge
          entry:
          bool_RpdDisChrgPerm = true;
          exit:
          bool_RpdDisChrgPerm = false;
        state BmsOff
          entry:
          st_BmsReq = uint8(BMSCmdTyp.BMS_CMD_HVOFF);
        state Motor_ShtDwn
        state HVAccStop
          entry:
          bool_DcDcEn = false;
          bool_AcPwrEnbl = false;
          bool_PtcPwrEnbl = false;
        state ChargerInit
          entry:
          st_ChrgrCmd = ChrgrCmdTyp.STOP;
          ChItCtr = 0;
          SlaveNoResponse = 0;
        Normal.HVOff.HV_OFF.HvOff_ERR -> Normal.HVOff.HV_OFF.HvOff : [V_MCU1MotCapVolt < pPUD_V_MotRpdDisVolt_C && ...
            | V_MCU2MotCapVolt < pPUD_V_MotRpdDisVolt_C ]
        Normal.HVOff.HV_OFF.RapidDischarge -> Normal.HVOff.HV_OFF.HvOff : [V_MCU1MotCapVolt < pPUD_V_MotRpdDisVolt_C && ...
            | V_MCU2MotCapVolt < pPUD_V_MotRpdDisVolt_C ]
        BmsOff -> Normal.HVOff.HV_OFF.RapidDischarge [order 1] : [st_BmsSts == BMSStsTyp.BMS_HVOFF_OK]
        BmsOff -> Normal.HVOff.HV_OFF.HvOff_ERR [order 2] : [st_BmsSts == BMSStsTyp.BMS_HVOFF_ERR]
        Normal.HVOff.HV_OFF.Motor_ShtDwn -> BmsOff : [bool_MotShtdwnAllow == true]
        HVAccStop -> Normal.HVOff.HV_OFF.Motor_ShtDwn : [st_DcDcActSts ==DCDCAStsTyp.DST_ShutDown && ...
            | bool_HvPwrOffEnbl == true || ...
            | after(pPUD_s_EgyCoorrNoRespTiout_C,sec)]
        Normal.HVOff.HV_OFF.ChargerInit -> HVAccStop : [st_ChrgrSts == ChrgrStsTyp.CST_STOP]
        (default) -> Normal.HVOff.HV_OFF.ChargerInit
      state Chrg_Check [parallel]
        settings: executionOrder=2
        (default) -> (junction 88)
        (junction 88) -> (junction 90) [order 2]
        (junction 88) -> (junction 91) [order 1] : [bool_ACChrgrPlugDtctd == false && ...
            | bool_DCChrgrPlugDtctd == false]
        (junction 91) -> (junction 92) : {
            | st_AcHeatModeSt = ACHeatModeTyp.PUD_ACHeat_Init;
            | st_ACChrgModeSt = ACChrgModeTyp.PUD_ACChrg_Init;
            | st_DCChrgModeSt = DCHeatModeTyp.PUD_DCHeat_Init;
            | st_DCChrgModeSt = DCChrgModeTyp.PUD_DCChrg_Init;
            | }
        (junction 90) -> (junction 93) [order 1] : [bool_ACChrgrPlugDtctd == false]
        (junction 93) -> (junction 94) : {
            | st_AcHeatModeSt = ACHeatModeTyp.PUD_ACHeat_Init;
            | st_ACChrgModeSt = ACChrgModeTyp.PUD_ACChrg_Init;
            | }
        (junction 92) -> (junction 94)
        (junction 98) -> (junction 89)
        (junction 97) -> (junction 89) [order 2]
        (junction 89) -> (junction 95)
        (junction 90) -> (junction 97) [order 2]
        (junction 97) -> (junction 96) [order 1] : [bool_DCChrgrPlugDtctd == false]
        (junction 94) -> (junction 98)
        (junction 96) -> (junction 98) : {
            | st_DCChrgModeSt = DCHeatModeTyp.PUD_DCHeat_Init;
            | st_DCChrgModeSt = DCChrgModeTyp.PUD_DCChrg_Init;
            | }
    state DCHeat
      settings: description=Charging control superstate.
      state DCHeat_Err
        entry:
        st_DCHeatModeSt = DCHeatModeTyp.PUD_DCHeat_Err;
        settings: description=Irrecoverable error state. This state is entered from any other state in the case of irrecoverable error and can only be left back into the HVoff state by resetting Clamp15 (ignition).
      state DCHeat_Init
        entry:
        st_ChrgrCmd = ChrgrCmdTyp.STOP;
        st_DCChrgModeSt = DCHeatModeTyp.PUD_DCHeat_Init;
        bool_DcDcEn = false;
        bool_AcPwrEnbl = false;
        bool_PtcPwrEnbl = false;
        ChItCtr = 0;
        SlaveNoResponse = 0;
      state DCHeat_On
        settings: description=Charging control superstate.
        state DCHeating
          settings: description=Charging control superstate.
          state Heating
            entry:
            st_DCHeatModeSt = DCHeatModeTyp.PUD_DCHeat_On;
            st_EgyCoorrSts = PUDCoorrStsTyp.PUD_DCHeatOn;
            settings: description=Normal charging operation. Charger mains maximum current and target voltage are set and charger is commanded to Active state on entry. Charger output current is computed dynamically according current BMS charging limitations. Start of charging is indicated acoustically by the buzzer.
          (default) -> Normal.DCHeat.DCHeat_On.DCHeating.Heating
          DCHeating -> DCHeating [order 1] : after(pPUD_s_EgyCoorrDlyRstCtr_C,sec)/ChItCtr = 0;
        state DcDcOKPtcOn
          entry:
          bool_PtcPwrEnbl = true;
        state BmsDCHeatOn
          entry:
          st_BmsReq = uint8(BMSCmdTyp.BMS_CMD_DCHeatOn);
        state BmsOkDcDcOn
          entry:
          bool_DcDcEn = true;
        state DCHeatPhase2
          entry:
          st_ChrgrCmd = uint8(ChrgrCmdTyp.DCHeat_PHASE2);
        state HVOFF
          entry:
          st_BmsReq = uint8(BMSCmdTyp.BMS_CMD_HVOFF);
        state DCHeatPhase1
          entry:
          st_ChrgrCmd = uint8(ChrgrCmdTyp.DCHeat_PHASE1);
        state DCHeatingInterrupted
          entry:
          ChItCtr = ChItCtr + 1;
          bool_DcDcEn = false;
          bool_AcPwrEnbl = false;
          bool_PtcPwrEnbl = false;
          st_ChrgrCmd = uint8(ChrgrCmdTyp.STOP);
        state ChargerInit
        DcDcOKPtcOn -> DCHeating
        Normal.DCHeat.DCHeat_On.HVOFF -> DCHeatPhase2 [order 1] : [st_BmsSts == BMSStsTyp.BMS_HVOFF_OK]
        DCHeating -> DCHeatingInterrupted [order 1] : [st_ChrgrSts == ChrgrStsTyp.CST_STOP]
        DCHeatPhase2 -> DCHeatingInterrupted [order 1] : after(pPUD_s_DCChrg2NoRespTiout_C,sec)
        DCHeatPhase2 -> BmsDCHeatOn [order 2] : [st_ChrgrSts == ChrgrStsTyp.CST_DCHeat_PHASE2]
        BmsDCHeatOn -> DCHeatingInterrupted [order 1] : after(pPUD_s_BMSOnNoRespTiout_C,sec)
        BmsDCHeatOn -> BmsOkDcDcOn [order 2] : [st_BmsSts == BMSStsTyp.BMS_DCHeatOn]
        BmsOkDcDcOn -> DCHeatingInterrupted [order 1] : after(pPUD_s_EgyCoorrNoRespTiout_C,sec)
        BmsOkDcDcOn -> DcDcOKPtcOn [order 2] : [st_DcDcActSts == DCDCAStsTyp.DST_Working]
        Normal.DCHeat.DCHeat_On.ChargerInit -> DCHeatPhase1
        DCHeatPhase1 -> DCHeatingInterrupted [order 1] : after(pPUD_s_DCChrg1NoRespTiout_C,sec)
        DCHeatPhase1 -> Normal.DCHeat.DCHeat_On.HVOFF [order 2] : [st_ChrgrSts == ChrgrStsTyp.CST_DCHeat_PHASE1]
        (default) -> Normal.DCHeat.DCHeat_On.ChargerInit
        DCHeatingInterrupted -> Normal.DCHeat.DCHeat_On.ChargerInit : after(pPUD_s_EgyCoorrChItRecoverDly_C,sec)
        Normal.DCHeat.DCHeat_On.HVOFF -> DCHeatingInterrupted [order 2] : after(pPUD_s_EgyCoorrNoRespTiout_C,sec)
      DCHeat_On -> DCHeat_Err : [ChItCtr > pPUD_cnt_DCHeatItErrThd_C]
      DCHeat_Init -> DCHeat_On
      (default) -> DCHeat_Init
    HVOff -> ACHeat [order 5] : [st_PUDCoorrReq == PUDCoorrStsTyp.PUD_ACHeatOn]
    DCChrg -> DCHeat [order 2] : [st_PUDCoorrReq == PUDCoorrStsTyp.PUD_DCHeatOn]
    Normal.Init -> HVOff [order 4] : [st_PUDCoorrReq == PUDCoorrStsTyp.PUD_HVOFF]
    HVOff -> DCHeat [order 4] : [st_PUDCoorrReq == PUDCoorrStsTyp.PUD_DCHeatOn]
    Normal.Init -> DCHeat [order 5] : [st_PUDCoorrReq == PUDCoorrStsTyp.PUD_DCHeatOn]
    ACHeat -> HVOff [order 1] : [st_PUDCoorrReq == PUDCoorrStsTyp.PUD_HVOFF]
    Normal.Init -> ACHeat [order 6] : [st_PUDCoorrReq == PUDCoorrStsTyp.PUD_ACHeatOn]
    DCHeat -> HVOff [order 1] : [st_PUDCoorrReq == PUDCoorrStsTyp.PUD_HVOFF]
    HVOff -> DCChrg [order 3] : [st_PUDCoorrReq == PUDCoorrStsTyp.PUD_DCChrgOn]
    HVOff -> Normal.ACChrg [order 1] : [st_PUDCoorrReq == PUDCoorrStsTyp.PUD_ACChrgOn]
    (default) -> Normal.Init
    Normal.Init -> Normal.ACChrg [order 3] : [st_PUDCoorrReq == PUDCoorrStsTyp.PUD_ACChrgOn]
    ACHeat -> Normal.ACChrg [order 2] : [st_PUDCoorrReq == PUDCoorrStsTyp.PUD_ACChrgOn]
    Normal.ACChrg -> HVOff [order 1] : [st_PUDCoorrReq == PUDCoorrStsTyp.PUD_HVOFF]
    DCHeat -> DCChrg [order 2] : [st_PUDCoorrReq == PUDCoorrStsTyp.PUD_DCChrgOn]
    Normal.Init -> DCChrg [order 2] : [st_PUDCoorrReq == PUDCoorrStsTyp.PUD_DCChrgOn]
    DCChrg -> HVOff [order 1] : [st_PUDCoorrReq == PUDCoorrStsTyp.PUD_HVOFF]
    Normal.Init -> Drv [order 1] : [st_PUDCoorrReq == PUDCoorrStsTyp.PUD_DrvOn]
      settings: description=Transit to HVon state of the BMS status changes to HVon.
    Drv -> HVOff : [st_PUDCoorrReq == PUDCoorrStsTyp.PUD_HVOFF]
      settings: description=Go to the HVoff state if BMS is in HVoff, Shutdown or Charging state. In case of charging, the machine will transit to the charging state through the HVOff state.
    HVOff -> Drv [order 2] : [st_PUDCoorrReq == PUDCoorrStsTyp.PUD_DrvOn]
    Normal.ACChrg -> ACHeat [order 2] : [st_PUDCoorrReq == PUDCoorrStsTyp.PUD_ACHeatOn]
  (default) -> Normal
  Normal -> EmgHVOff : [st_PUDCoorrReq == PUDCoorrStsTyp.PUD_EmgHVOFF]
  data: st_PUDCoorrReq input double; bool_MotShtdwnAllow input double; V_MCU1MotCapVolt input double; V_MCU2MotCapVolt input double; bool_HvPwrOffEnbl input double; bool_ACChrgrPlugDtctd input double; bool_DCChrgrPlugDtctd input double; st_BmsSts input double; st_ChrgrSts input double; st_DcDcActSts input double; st_EgyCoorrSts output uint8 =PUDCoorrStsTyp.PUD_HVOFF; st_BmsReq output uint8 =BMSCmdTyp.BMS_CMD_IDLE; st_ChrgrCmd output uint8; bool_DcDcEn output boolean =0; SlaveNoResponse local boolean =0; pPUD_s_EgyCoorrNoRespTiout_C input single =0.5; ChItCtr local uint8; pPUD_s_EgyCoorrChItRecoverDly_C input double; pPUD_s_EgyCoorrDlyRstCtr_C input double; bool_AcPwrEnbl output boolean; st_ACChrgModeSt output uint8; st_DCChrgModeSt output uint8; st_AcHeatModeSt output uint8; st_DCHeatModeSt output uint8; st_DrvOnModeSt output uint8; bool_PtcPwrEnbl output boolean; bool_RpdDisChrgPerm output boolean; pPUD_V_MotRpdDisVolt_C input double; pPUD_s_DCChrg1NoRespTiout_C input double; pPUD_s_BMSOnNoRespTiout_C input double; pPUD_s_ACChrg1NoRespTiout_C input double; pPUD_s_ACChrg2NoRespTiout_C input double; pPUD_s_DCChrg2NoRespTiout_C input double; pPUD_cnt_ACChItErrThd_C input double; pPUD_cnt_DCChItErrThd_C input double; pPUD_cnt_ACHeatItErrThd_C input double; pPUD_cnt_DCHeatItErrThd_C input double; pPUD_V_MotPwrVolt_C input double; pPUD_s_ACChrgPtcEnDly_C input double
